simulink model "project"  (R2023a)
settings: Solver=VariableStepAuto  StartTime=0.0  StopTime=100  RelTol=1e-3
libraries: slpidlib x1
settings Model: PacingRate=0.790000  Creator=itsma  LastModifiedBy=itsma

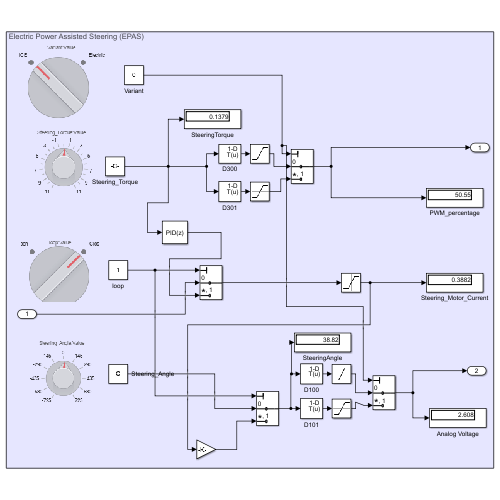
[thumbnail: Simulink's stored preview of the top-level diagram]
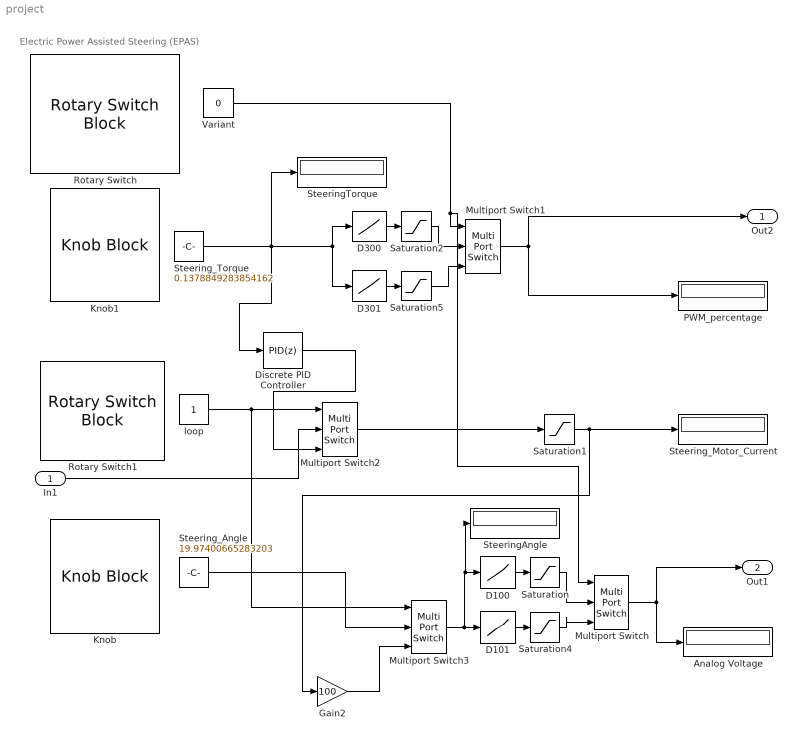
== system project ==
  note: Electric Power Assisted Steering (EPAS)
  In1 : Inport
  Analog Voltage : Display
  D100 : Lookup_n-D  NumberOfTableDimensions=1  BreakpointsForDimension1=[-720.1;-720;0;720;720.1]  Table=[0;0.5;2.5;4.5;5]  InternalRulePriority=Speed  RndMeth=Simplest
  D101 : Lookup_n-D  NumberOfTableDimensions=1  BreakpointsForDimension1=[-720.1;-720;720;720.1]  Table=[0;1;9;10]  InternalRulePriority=Speed  RndMeth=Simplest
  D300 : Lookup_n-D  NumberOfTableDimensions=1  BreakpointsForDimension1=[-10.01;-10;10;10.01]  Table=[0;10;90;100]  InternalRulePriority=Speed  RndMeth=Simplest
  D301 : Lookup_n-D  NumberOfTableDimensions=1  BreakpointsForDimension1=[-10.01;-10;10;10.01]  Table=[0;3;97;10]  InternalRulePriority=Speed  RndMeth=Simplest
  Discrete PID Controller : slpidlib/PID Controller  Controller=PID  Form=Parallel  TimeDomain=Discrete-time  UseExternalTs=off  SampleTime=-1  IntegratorMethod=Forward Euler  FilterMethod=Forward Euler  ControllerParametersSource=internal  P=0.25  I=0.1  UseKiTs=off  D=0  N=100  UseFilter=on  TunerSelectOption=Transfer Function Based (PID Tuner App)  InitialConditionSource=internal  InitialConditionForIntegrator=0  InitialConditionForFilter=0  DifferentiatorICPrevScaledInput=0  ExternalReset=none  TrackingMode=off  Kt=1  LimitOutput=off  SatLimitsSource=internal  UpperSaturationLimit=inf  LowerSaturationLimit=-inf  LinearizeAsGain=off  AntiWindupMode=none  Kb=1  LimitIntegrator=off  UpperIntegratorSaturationLimit=inf  LowerIntegratorSaturationLimit=-inf  POutMin=[]  POutMax=[]  IOutMin=[]  IOutMax=[]  DOutMin=[]  DOutMax=[]  NOutMin=[]  NOutMax=[]  SumOutMin=[]  SumOutMax=[]  SaturationOutMin=[]  SaturationOutMax=[]  PParamMin=[]  PParamMax=[]  IParamMin=[]  IParamMax=[]  DParamMin=[]  DParamMax=[]  NParamMin=[]  NParamMax=[]  KbParamMin=[]  KbParamMax=[]  KtParamMin=[]  KtParamMax=[]  KbOutMin=[]  KbOutMax=[]  KtOutMin=[]  KtOutMax=[]  IntegratorOutMin=[]  IntegratorOutMax=[]  FilterOutMin=[]  FilterOutMax=[]  SumI1OutMin=[]  SumI1OutMax=[]  SumI2OutMin=[]  SumI2OutMax=[]  SumI3OutMin=[]  SumI3OutMax=[]  SumI4OutMin=[]  SumI4OutMax=[]  SumDOutMin=[]  SumDOutMax=[]  DifferentiatorOutMin=[]  DifferentiatorOutMax=[]  FilterDiffOutCoefMin=[]  FilterDiffOutCoefMax=[]  ReciprocalOutMin=[]  ReciprocalOutMax=[]  SumDenOutMin=[]  SumDenOutMax=[]  SumNumOutMin=[]  SumNumOutMax=[]  DivideOutMin=[]  DivideOutMax=[]  UdiffTsProdOutMin=[]  UdiffTsProdOutMax=[]  NTsProdOutMin=[]  NTsProdOutMax=[]  UintegralTsProdOutMin=[]  UintegralTsProdOutMax=[]  UngainTsProdOutMin=[]  UngainTsProdOutMax=[]  ClampingZeroOutDataTypeStr=Inherit: Inherit via back propagation  ClampingZeroOutMin=[]  ClampingZeroOutMax=[]  FilterDenConstantOutDataTypeStr=Inherit: Inherit via back propagation  FilterDenConstantOutMin=[]  FilterDenConstantOutMax=[]  PCopyOutDataTypeStr=Inherit: Inherit via back propagation  PCopyOutMin=[]  PCopyOutMax=[]  NCopyOutDataTypeStr=Inherit: Inherit via back propagation  NCopyOutMin=[]  NCopyOutMax=[]  IntegratorContinuousStateAttributes=''  IntegratorStateMustResolveToSignalObject=off  IntegratorRTWStateStorageClass=Auto  FilterContinuousStateAttributes=''  FilterStateMustResolveToSignalObject=off  FilterRTWStateStorageClass=Auto  ParallelPVariant=InternalParameters  IdealPVariant=Disabled  IVariant=InternalParameters  DVariant=InternalParameters  IntegratorVariant=Discrete  SatVariant=Disabled  AWVariant=Passthrough  PCopyVariant=Disabled  TRVariant=Disabled  FdbkBlocksVariant=Forward  IdealPFdbkVariant=Disabled  SatFdbkVariant=Disabled  DerivativeFilterVariant=ForwardEulerFilter  NVariant=InternalParameters  NCopyVariant=Disabled  FilterICVariant=InternalICsFilter  IntegratorICVariant=InternalICs  ExternalResetVariant=Disabled  TRSumVariant=Passthrough  SumFdbkVariant=Disabled  SumVariant=Sum_PID  TsampFilterVariant=InternalTs  TsampNgainVariant=Passthrough  TsampIntegralVariant=Disabled_SignalSpec  ExternalSaturationOutDataTypeStr=Inherit: Same as second input
      settings: LibrarySourceBlock=simulink/Discrete/Discrete PID Controller
  Gain2 : Gain  Gain=100
  Knob : KnobBlock  ScaleMin=-725  ScaleMax=725
  Knob1 : KnobBlock  ScaleMin=-11  ScaleMax=11
  Multiport Switch{,1..3} (4 alike) : MultiPortSwitch  DataPortOrder=Zero-based contiguous  Inputs=2  zeroidx=on  SaturateOnIntegerOverflow=off  InputSameDT=off
  PWM_percentage : Display
  Rotary Switch : RotarySwitchBlock
      settings: Values={{'ICE', 'Electric'}, [0 1]}
  Rotary Switch1 : RotarySwitchBlock
      settings: Values={{'Open', 'Closed'}, [0 1]}
  Saturation : Saturate  UpperLimit=5  LowerLimit=0
  Saturation1 : Saturate  UpperLimit=6  LowerLimit=-6
  Saturation2 : Saturate  UpperLimit=100  LowerLimit=0
  Saturation4 : Saturate  UpperLimit=10  LowerLimit=0
  Saturation5 : Saturate  UpperLimit=100  LowerLimit=0
  SteeringAngle : Display
  SteeringTorque : Display
  Steering_Angle : Constant  Value=19.97400665283203
  Steering_Motor_Current : Display
  Steering_Torque : Constant  Value=0.1378849283854162
  Variant : Constant  Value=0
  loop : Constant
  Out2 : Outport
  Out1 : Outport  Port=2
  wires:
  Multiport Switch/1 -> Out1/1, Analog Voltage/1
  Saturation4/1 -> Multiport Switch/3
  Multiport Switch3/1 -> SteeringAngle/1, D100/1, D101/1
  Steering_Torque/1 -> Discrete PID Controller/1, D301/1, D300/1, SteeringTorque/1
  Saturation2/1 -> Multiport Switch1/2
  Discrete PID Controller/1 -> Multiport Switch2/3
  D101/1 -> Saturation4/1
  loop/1 -> Multiport Switch3/1, Multiport Switch2/1
  Multiport Switch1/1 -> Out2/1, PWM_percentage/1
  Variant/1 -> Multiport Switch/1, Multiport Switch1/1
  Saturation/1 -> Multiport Switch/2
  Multiport Switch2/1 -> Saturation1/1
  Saturation1/1 -> Gain2/1, Steering_Motor_Current/1
  D300/1 -> Saturation2/1
  Saturation5/1 -> Multiport Switch1/3
  D301/1 -> Saturation5/1
  Gain2/1 -> Multiport Switch3/3
  D100/1 -> Saturation/1
  Steering_Angle/1 -> Multiport Switch3/2
  In1/1 -> Multiport Switch2/2
